simulink model "c_code_MR100"  (R2023a)
settings: Solver=FixedStepAuto  StartTime=0.0  StopTime=10  FixedStep=0.01  MaxStep=0.01  RelTol=1e-3
settings Model: Creator=LJL  LastModifiedBy=LJL
settings OptimizationCC: DefaultParameterBehavior=Inlined  UseDivisionForNetSlopeComputation=on  GainParamInheritBuiltInType=on  UseFloatMulNetSlope=on  InlineInvariantSignals=on  EnhancedBackFolding=on  BooleansAsBitfields=on  PassReuseOutputArgsAs=Individual arguments  StateBitsets=on  DataBitsets=on  ZeroExternalMemoryAtStartup=off  ZeroInternalMemoryAtStartup=off  NoFixptDivByZeroProtection=on  EfficientFloat2IntCast=on  LifeSpan=1  OptimizeBlockOrder=speed  DifferentSizesBufferReuse=on  EfficientTunableParamExpr=on
settings DebuggingCC: ParameterTunabilityLossMsg=error
settings HardwareCC: ProdBitPerInt=16  ProdBitPerPointer=16  ProdBitPerSizeT=16  ProdBitPerPtrDiffT=16  ProdLargestAtomicFloat=None  ProdWordSize=16  ProdLongLongMode=on  ProdHWDeviceType=STMicroelectronics->ST10/Super10
settings SFSimCC: MATLABDynamicMemAlloc=off
settings RTWCC: Description=Embedded Coder  SystemTargetFile=ert.tlc  PackageGeneratedCodeAndArtifacts=on  TemplateMakefile=ert_default_tmf  GenerateReport=on  IncludeHyperlinkInReport=on  LaunchReport=on  GenerateTraceInfo=on  GenerateTraceReport=on  GenerateTraceReportSl=on  GenerateWebview=on
settings CodeAppCC: ForceParamTrailComments=on  IgnoreCustomStorageClasses=off  OperatorAnnotations=on  SimulinkDataObjDesc=on  SFDataObjDesc=on  CustomSymbolStrGlobalVar=rt$N$M  CustomSymbolStrType=$N$M  CustomSymbolStrFcn=$N$M$F  CustomSymbolStrMacro=$N$M  InsertBlockDesc=on
settings ERTTargetCC: TargetLangStandard=C99 (ISO)  GenerateSampleERTMain=on  IncludeMdlTerminateFcn=off  CombineSignalStateStructs=on  SupportComplex=off  SupportContinuousTime=on  InlinedParameterPlacement=NonHierarchical  ERTCustomFileTemplate=example_file_process.tlc  ERTFilePackagingFormat=CompactWithDataFile

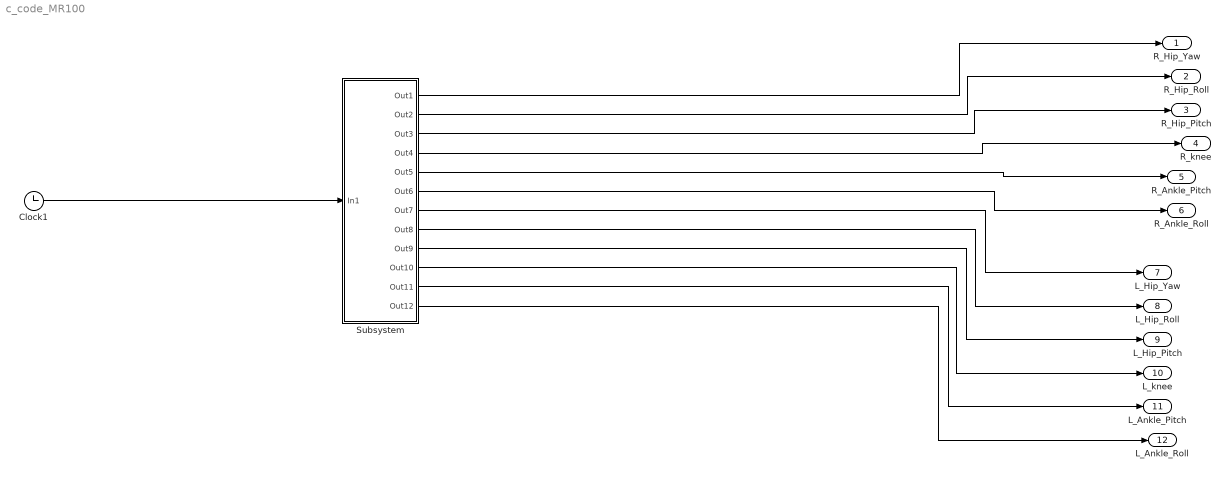
== system c_code_MR100 ==
  Clock1 : Clock
      settings: Decimation=5
  Subsystem : Subsystem
  R_Hip_Yaw : Outport
  R_Hip_Roll : Outport  Port=2
  R_Hip_Pitch : Outport  Port=3
  R_knee : Outport  Port=4
  R_Ankle_Pitch : Outport  Port=5
  R_Ankle_Roll : Outport  Port=6
  L_Hip_Yaw : Outport  Port=7
  L_Hip_Roll : Outport  Port=8
  L_Hip_Pitch : Outport  Port=9
  L_knee : Outport  Port=10
  L_Ankle_Pitch : Outport  Port=11
  L_Ankle_Roll : Outport  Port=12
  wires:
  Clock1/1 -> Subsystem/1(In1)
  Subsystem/1(Out1) -> R_Hip_Yaw/1
  Subsystem/2(Out2) -> R_Hip_Roll/1
  Subsystem/3(Out3) -> R_Hip_Pitch/1
  Subsystem/4(Out4) -> R_knee/1
  Subsystem/5(Out5) -> R_Ankle_Pitch/1
  Subsystem/6(Out6) -> R_Ankle_Roll/1
  Subsystem/7(Out7) -> L_Hip_Yaw/1
  Subsystem/8(Out8) -> L_Hip_Roll/1
  Subsystem/9(Out9) -> L_Hip_Pitch/1
  Subsystem/10(Out10) -> L_knee/1
  Subsystem/11(Out11) -> L_Ankle_Pitch/1
  Subsystem/12(Out12) -> L_Ankle_Roll/1

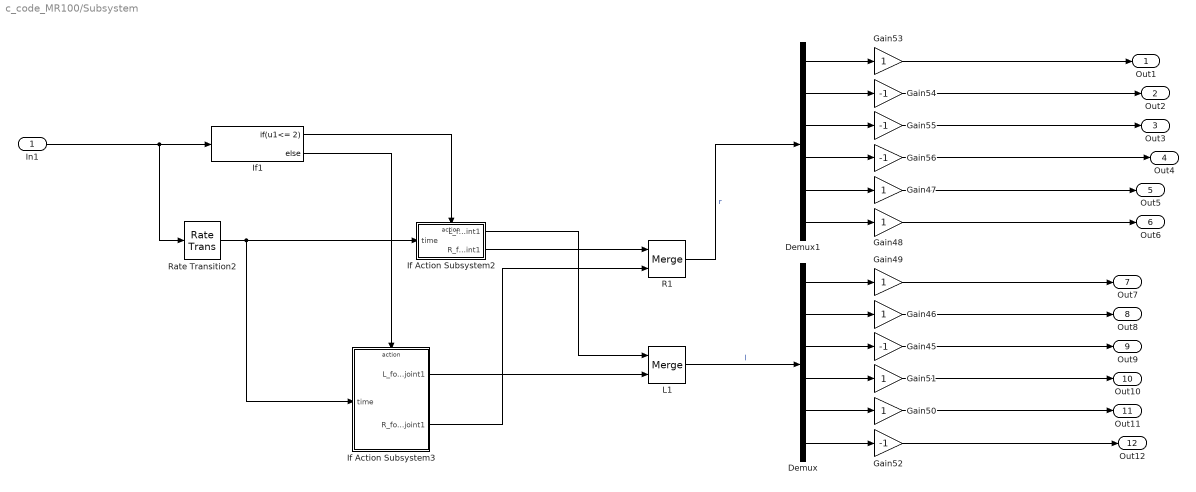
== system c_code_MR100/Subsystem ==
  In1 : Inport
  Demux : Demux  Outputs=6
  Demux1 : Demux  Outputs=6
  Gain{45,52,54..56} (5 alike) : Gain  Gain=-1
  Gain{46..51,53} (7 alike) : Gain
  If Action Subsystem2 : Subsystem  TreatAsAtomicUnit=on
  If Action Subsystem3 : Subsystem  TreatAsAtomicUnit=on
  If1 : If  IfExpression=u1<= 2
  L1 : Merge
  R1 : Merge
  Rate Transition2 : RateTransition  OutPortSampleTime=0.01
  Out1 : Outport
  Out2 : Outport  Port=2
  Out3 : Outport  Port=3
  Out4 : Outport  Port=4
  Out5 : Outport  Port=5
  Out6 : Outport  Port=6
  Out7 : Outport  Port=7
  Out8 : Outport  Port=8
  Out9 : Outport  Port=9
  Out10 : Outport  Port=10
  Out11 : Outport  Port=11
  Out12 : Outport  Port=12
  wires:
  Demux/1 -> Gain49/1
  Demux1/2 -> Gain54/1
  If Action Subsystem2/2(R_foot_joint1) -> R1/1
  Gain52/1 -> Out12/1
  Demux/4 -> Gain51/1
  Demux/6 -> Gain52/1
  Demux/5 -> Gain50/1
  In1/1 -> Rate Transition2/1, If1/1
  If Action Subsystem3/2(R_foot_joint1) -> R1/2
  Rate Transition2/1 -> If Action Subsystem3/1(time), If Action Subsystem2/1(time)
  Demux/2 -> Gain46/1
  If Action Subsystem2/1(L_foot_joint1) -> L1/1
  Demux/3 -> Gain45/1
  Gain46/1 -> Out8/1
  Demux1/3 -> Gain55/1
  Demux1/4 -> Gain56/1
  L1/1 -> Demux/1  "l"
  If1/1 -> If Action Subsystem2/Action
  Demux1/1 -> Gain53/1
  Gain50/1 -> Out11/1
  Demux1/5 -> Gain47/1
  Gain48/1 -> Out6/1
  Demux1/6 -> Gain48/1
  R1/1 -> Demux1/1  "r"
  Gain55/1 -> Out3/1
  If1/2 -> If Action Subsystem3/Action
  Gain54/1 -> Out2/1
  If Action Subsystem3/1(L_foot_joint1) -> L1/2
  Gain56/1 -> Out4/1
  Gain51/1 -> Out10/1
  Gain53/1 -> Out1/1
  Gain47/1 -> Out5/1
  Gain49/1 -> Out7/1
  Gain45/1 -> Out9/1

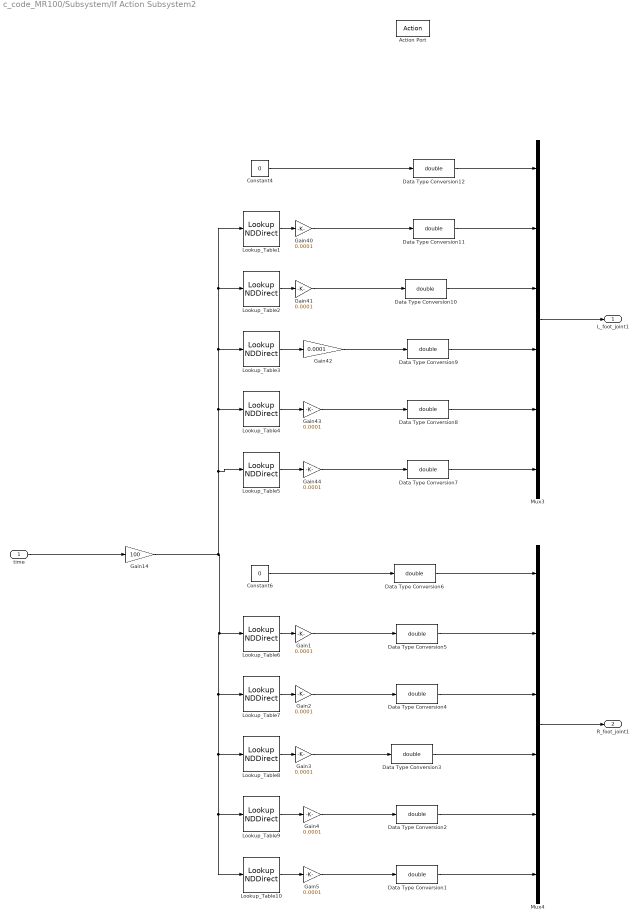
== system c_code_MR100/Subsystem/If Action Subsystem2 ==
  time : Inport
  Action Port : ActionPort  ActionPortLabel=if(u1<= 2)
  Constant4 : Constant  Value=0  SampleTime=-1
  Constant6 : Constant  Value=0  SampleTime=-1
  Data Type Conversion{1..12} (12 alike) : DataTypeConversion  OutDataTypeStr=double  SaturateOnIntegerOverflow=off  RndMeth=Floor
  Gain{1..5,40..44} (10 alike) : Gain  Gain=0.0001
  Gain14 : Gain  Gain=100
  Lookup_Table1 : LookupNDDirect  NumberOfTableDimensions=1  Table=[0;0;0;0;0;0;0;0;0;0;0;0;0;0;0;0;0;0;0;0;0;0;0;0;0;0;0;0;0;0;0;0;0;0;0;0;0;0;0;0;0;0;0;0;0;0;0;0;0;0;0;0;0;0;0;0;0;0;0;0;0;0;0;0;0;0;0;0;0;0;0;0;0;0;0;0;0;0;0;0;0;0;0;0;0;0;0;0;0;0;0;0;0;0;0;0;0;0;0;0;0;0;0;0;0;-1;-1;-2;-4;-6;-9;-12;-17;-22;-29;-37;-46;-57;-69;-83;-99;-117;-137;-159;-183;-209;-238;-269;-303;-339;-378;-420;-463;-510;-559;-610;-664;-720;-779;-839;-902;-966;-1032;-1100;-1169;-1238;-1309;-1380;-1451;-1523;-1593;-1664;-1733;-1802;-1873;-1945;-2018;-2091;-2165;-2238;-2311;-2382;-2452;-2519;-2584;-2644;-2700;-2751;-2795;-2832;-2861;-2882;-2892;-2892;-2881;-2857;-2824;-2781;-2725;-2658;-2580;-2493;-2397;-2294;-2183;-2067;-1946;-1821;-1693;-1562;-1428;-1293;-1157;-1020;-882;-744;-605;-466;-327;-187;-47]  RemoveProtectionInput=on  TableDataTypeStr=int16
  Lookup_Table10 : LookupNDDirect  NumberOfTableDimensions=1  Table=[0;0;0;0;0;0;0;0;0;0;0;0;0;0;0;0;0;0;0;0;0;0;0;0;0;0;0;0;0;0;0;0;0;0;0;0;0;0;0;0;0;0;0;0;0;0;0;0;0;0;0;0;0;0;0;0;0;0;0;0;0;0;0;0;0;0;0;0;0;0;0;0;0;0;0;0;0;0;0;0;0;0;0;0;0;0;0;0;0;0;0;0;0;0;0;0;0;0;0;0;0;0;0;0;0;1;1;2;4;6;9;12;17;22;29;37;46;57;69;83;99;117;137;159;183;209;238;269;303;339;378;420;463;510;559;610;664;720;779;839;902;966;1032;1100;1169;1238;1309;1380;1451;1523;1593;1664;1733;1801;1867;1931;1993;2053;2110;2163;2214;2260;2303;2342;2377;2407;2433;2454;2470;2481;2486;2486;2481;2470;2453;2430;2401;2367;2326;2279;2226;2166;2101;2029;1951;1867;1777;1682;1581;1474;1362;1246;1124;999;870;738;603;466;327;187;47]  RemoveProtectionInput=on  TableDataTypeStr=int16
  Lookup_Table2 : LookupNDDirect  NumberOfTableDimensions=1  Table=[0;0;0;0;0;0;0;0;0;0;0;0;0;0;0;0;0;0;0;0;0;0;0;0;0;0;0;0;0;0;0;0;0;0;0;0;0;0;0;0;0;0;0;0;0;0;0;0;0;0;223;277;396;536;683;832;981;1128;1274;1418;1560;1699;1837;1971;2103;2233;2360;2484;2606;2724;2840;2953;3063;3170;3273;3374;3472;3566;3657;3745;3830;3911;3989;4063;4134;4201;4264;4324;4380;4432;4480;4524;4564;4600;4631;4658;4681;4698;4711;4719;4719;4719;4719;4719;4719;4719;4719;4719;4719;4719;4719;4719;4719;4719;4719;4719;4719;4719;4719;4719;4718;4718;4718;4717;4717;4716;4716;4715;4713;4712;4710;4708;4706;4703;4700;4696;4692;4687;4682;4676;4669;4662;4654;4645;4635;4624;4613;4601;4588;4574;4560;4545;4530;4524;4538;4568;4614;4671;4739;4816;4898;4984;5072;5161;5249;5335;5418;5495;5567;5633;5692;5742;5783;5815;5835;5845;5848;5846;5830;5803;5766;5719;5663;5599;5529;5452;5372;5287;5201;5114;5029;4946;4869;4799;4738;4689;4655;4637;4638;4648;4655]  RemoveProtectionInput=on  TableDataTypeStr=int16
  Lookup_Table3 : LookupNDDirect  NumberOfTableDimensions=1  Table=[0;0;0;0;0;0;0;0;0;0;0;0;0;0;0;0;0;0;0;0;0;0;0;0;0;0;0;0;0;0;0;0;0;0;0;0;0;0;0;0;0;0;0;0;0;0;0;0;0;0;552;688;983;1332;1697;2067;2437;2805;3169;3528;3883;4233;4578;4917;5250;5577;5899;6214;6523;6826;7123;7412;7695;7972;8241;8503;8758;9005;9244;9476;9700;9916;10123;10322;10511;10692;10864;11026;11178;11320;11452;11573;11683;11781;11868;11943;12005;12054;12090;12112;12112;12112;12112;12112;12112;12112;12112;12112;12112;12112;12112;12112;12112;12112;12112;12112;12112;12112;12111;12111;12110;12110;12109;12108;12106;12105;12103;12100;12097;12093;12088;12082;12076;12068;12059;12049;12037;12024;12009;11992;11974;11953;11930;11905;11878;11849;11817;11784;11748;11711;11671;11631;11588;11573;11611;11694;11819;11980;12169;12382;12614;12858;13110;13366;13622;13873;14117;14349;14566;14766;14944;15100;15228;15326;15392;15420;15432;15424;15376;15291;15174;15028;14856;14662;14449;14221;13981;13733;13482;13231;12986;12751;12532;12335;12165;12029;11933;11884;11887;11914;11934]  RemoveProtectionInput=on  TableDataTypeStr=int16
  Lookup_Table4 : LookupNDDirect  NumberOfTableDimensions=1  Table=[0;0;0;0;0;0;0;0;0;0;0;0;0;0;0;0;0;0;0;0;0;0;0;0;0;0;0;0;0;0;0;0;0;0;0;0;0;0;0;0;0;0;0;0;0;0;0;0;0;0;330;411;587;795;1014;1235;1456;1676;1895;2110;2323;2534;2741;2945;3146;3344;3539;3730;3918;4102;4283;4460;4633;4802;4967;5129;5286;5439;5587;5731;5870;6005;6134;6259;6378;6491;6599;6702;6798;6888;6972;7048;7119;7181;7237;7285;7324;7356;7379;7393;7393;7393;7393;7393;7393;7393;7393;7393;7393;7393;7393;7393;7393;7393;7393;7393;7393;7393;7393;7392;7392;7392;7391;7390;7389;7388;7387;7385;7383;7381;7378;7374;7370;7365;7359;7353;7345;7337;7327;7316;7304;7291;7277;7261;7243;7225;7204;7183;7160;7136;7111;7085;7059;7049;7073;7126;7206;7308;7430;7567;7716;7874;8038;8205;8373;8538;8699;8853;8998;9132;9253;9358;9445;9512;9556;9576;9584;9578;9545;9488;9408;9309;9193;9063;8920;8768;8609;8446;8281;8117;7957;7805;7663;7536;7427;7340;7278;7247;7249;7266;7279]  RemoveProtectionInput=on  TableDataTypeStr=int16
  Lookup_Table5 : LookupNDDirect  NumberOfTableDimensions=1  Table=[0;0;0;0;0;0;0;0;0;0;0;0;0;0;0;0;0;0;0;0;0;0;0;0;0;0;0;0;0;0;0;0;0;0;0;0;0;0;0;0;0;0;0;0;0;0;0;0;0;0;0;0;0;0;0;0;0;0;0;0;0;0;0;0;0;0;0;0;0;0;0;0;0;0;0;0;0;0;0;0;0;0;0;0;0;0;0;0;0;0;0;0;0;0;0;0;0;0;0;0;0;0;0;0;0;1;1;2;4;6;9;12;17;22;29;37;46;57;69;83;99;117;137;159;183;209;238;269;303;339;378;420;463;510;559;610;664;720;779;839;902;966;1032;1100;1169;1238;1309;1380;1451;1523;1593;1664;1733;1802;1873;1945;2018;2091;2165;2238;2311;2382;2452;2519;2584;2644;2700;2751;2795;2832;2861;2882;2892;2892;2881;2857;2824;2781;2725;2658;2580;2493;2397;2294;2183;2067;1946;1821;1693;1562;1428;1293;1157;1020;882;744;605;466;327;187;47]  RemoveProtectionInput=on  TableDataTypeStr=int16
  Lookup_Table6 : LookupNDDirect  NumberOfTableDimensions=1  Table=[0;0;0;0;0;0;0;0;0;0;0;0;0;0;0;0;0;0;0;0;0;0;0;0;0;0;0;0;0;0;0;0;0;0;0;0;0;0;0;0;0;0;0;0;0;0;0;0;0;0;0;0;0;0;0;0;0;0;0;0;0;0;0;0;0;0;0;0;0;0;0;0;0;0;0;0;0;0;0;0;0;0;0;0;0;0;0;0;0;0;0;0;0;0;0;0;0;0;0;0;0;0;0;0;0;-1;-1;-2;-4;-6;-9;-12;-17;-22;-29;-37;-46;-57;-69;-83;-99;-117;-137;-159;-183;-209;-238;-269;-303;-339;-378;-420;-463;-510;-559;-610;-664;-720;-779;-839;-902;-966;-1032;-1100;-1169;-1238;-1309;-1380;-1451;-1523;-1593;-1664;-1733;-1801;-1867;-1931;-1993;-2053;-2110;-2163;-2214;-2260;-2303;-2342;-2377;-2407;-2433;-2454;-2470;-2481;-2486;-2486;-2481;-2470;-2453;-2430;-2401;-2367;-2326;-2279;-2226;-2166;-2101;-2029;-1951;-1867;-1777;-1682;-1581;-1474;-1362;-1246;-1124;-999;-870;-738;-603;-466;-327;-187;-47]  RemoveProtectionInput=on  TableDataTypeStr=int16
  Lookup_Table7 : LookupNDDirect  NumberOfTableDimensions=1  Table=[0;0;0;0;0;0;0;0;0;0;0;0;0;0;0;0;0;0;0;0;0;0;0;0;0;0;0;0;0;0;0;0;0;0;0;0;0;0;0;0;0;0;0;0;0;0;0;0;0;0;223;277;396;536;683;832;981;1128;1274;1418;1560;1699;1837;1971;2103;2233;2360;2484;2606;2724;2840;2953;3063;3170;3273;3374;3472;3566;3657;3745;3830;3911;3989;4063;4134;4201;4264;4324;4380;4432;4480;4524;4564;4600;4631;4658;4681;4698;4711;4719;4719;4719;4719;4719;4719;4719;4719;4719;4719;4719;4719;4719;4719;4719;4719;4719;4719;4719;4719;4719;4718;4718;4718;4717;4717;4716;4716;4715;4713;4712;4710;4708;4706;4703;4700;4696;4692;4687;4682;4676;4669;4662;4654;4645;4635;4624;4613;4601;4588;4574;4560;4545;4530;4514;4498;4482;4466;4449;4433;4418;4403;4388;4375;4362;4350;4340;4331;4324;4319;4315;4313;4312;4314;4318;4323;4331;4340;4352;4365;4379;4395;4412;4430;4449;4469;4489;4509;4529;4549;4568;4586;4603;4618;4632;4644;4654;4661;4666;4669;4669;4667]  RemoveProtectionInput=on  TableDataTypeStr=int16
  Lookup_Table8 : LookupNDDirect  NumberOfTableDimensions=1  Table=[0;0;0;0;0;0;0;0;0;0;0;0;0;0;0;0;0;0;0;0;0;0;0;0;0;0;0;0;0;0;0;0;0;0;0;0;0;0;0;0;0;0;0;0;0;0;0;0;0;0;552;688;983;1332;1697;2067;2437;2805;3169;3528;3883;4233;4578;4917;5250;5577;5899;6214;6523;6826;7123;7412;7695;7972;8241;8503;8758;9005;9244;9476;9700;9916;10123;10322;10511;10692;10864;11026;11178;11320;11452;11573;11683;11781;11868;11943;12005;12054;12090;12112;12112;12112;12112;12112;12112;12112;12112;12112;12112;12112;12112;12112;12112;12112;12112;12112;12112;12112;12111;12111;12110;12110;12109;12108;12106;12105;12103;12100;12097;12093;12088;12082;12076;12068;12059;12049;12037;12024;12009;11992;11974;11953;11930;11905;11878;11849;11817;11784;11748;11711;11671;11631;11588;11545;11501;11457;11412;11368;11324;11281;11240;11200;11163;11129;11098;11070;11046;11026;11011;11000;10995;10994;10999;11009;11024;11045;11070;11101;11136;11175;11218;11265;11315;11367;11421;11476;11531;11586;11640;11693;11743;11789;11832;11870;11903;11930;11951;11966;11973;11973;11966]  RemoveProtectionInput=on  TableDataTypeStr=int16
  Lookup_Table9 : LookupNDDirect  NumberOfTableDimensions=1  Table=[0;0;0;0;0;0;0;0;0;0;0;0;0;0;0;0;0;0;0;0;0;0;0;0;0;0;0;0;0;0;0;0;0;0;0;0;0;0;0;0;0;0;0;0;0;0;0;0;0;0;330;411;587;795;1014;1235;1456;1676;1895;2110;2323;2534;2741;2945;3146;3344;3539;3730;3918;4102;4283;4460;4633;4802;4967;5129;5286;5439;5587;5731;5870;6005;6134;6259;6378;6491;6599;6702;6798;6888;6972;7048;7119;7181;7237;7285;7324;7356;7379;7393;7393;7393;7393;7393;7393;7393;7393;7393;7393;7393;7393;7393;7393;7393;7393;7393;7393;7393;7393;7392;7392;7392;7391;7390;7389;7388;7387;7385;7383;7381;7378;7374;7370;7365;7359;7353;7345;7337;7327;7316;7304;7291;7277;7261;7243;7225;7204;7183;7160;7136;7111;7085;7059;7031;7003;6975;6946;6918;6890;6863;6837;6812;6789;6767;6747;6730;6714;6702;6692;6686;6682;6682;6685;6691;6701;6714;6730;6749;6771;6796;6824;6853;6885;6918;6952;6987;7022;7057;7092;7125;7157;7187;7214;7238;7259;7277;7290;7299;7304;7304;7300]  RemoveProtectionInput=on  TableDataTypeStr=int16
  Mux3 : Mux  Inputs=6
  Mux4 : Mux  Inputs=6
  L_foot_joint1 : Outport
  R_foot_joint1 : Outport  Port=2
  wires:
  Constant4/1 -> Data Type Conversion12/1
  Lookup_Table4/1 -> Gain43/1
  Lookup_Table3/1 -> Gain42/1
  Lookup_Table5/1 -> Gain44/1
  Lookup_Table1/1 -> Gain40/1
  time/1 -> Gain14/1
  Lookup_Table2/1 -> Gain41/1
  Mux3/1 -> L_foot_joint1/1
  Gain43/1 -> Data Type Conversion8/1
  Gain42/1 -> Data Type Conversion9/1
  Gain44/1 -> Data Type Conversion7/1
  Gain41/1 -> Data Type Conversion10/1
  Gain40/1 -> Data Type Conversion11/1
  Gain1/1 -> Data Type Conversion5/1
  Gain2/1 -> Data Type Conversion4/1
  Lookup_Table7/1 -> Gain2/1
  Gain5/1 -> Data Type Conversion1/1
  Lookup_Table9/1 -> Gain4/1
  Lookup_Table6/1 -> Gain1/1
  Lookup_Table10/1 -> Gain5/1
  Lookup_Table8/1 -> Gain3/1
  Gain3/1 -> Data Type Conversion3/1
  Gain4/1 -> Data Type Conversion2/1
  Mux4/1 -> R_foot_joint1/1
  Gain14/1 -> Lookup_Table7/1, Lookup_Table8/1, Lookup_Table9/1, Lookup_Table10/1, Lookup_Table6/1, Lookup_Table5/1, Lookup_Table1/1, Lookup_Table2/1, Lookup_Table3/1, Lookup_Table4/1
  Constant6/1 -> Data Type Conversion6/1
  Data Type Conversion1/1 -> Mux4/6
  Data Type Conversion2/1 -> Mux4/5
  Data Type Conversion3/1 -> Mux4/4
  Data Type Conversion4/1 -> Mux4/3
  Data Type Conversion5/1 -> Mux4/2
  Data Type Conversion6/1 -> Mux4/1
  Data Type Conversion7/1 -> Mux3/6
  Data Type Conversion8/1 -> Mux3/5
  Data Type Conversion9/1 -> Mux3/4
  Data Type Conversion10/1 -> Mux3/3
  Data Type Conversion11/1 -> Mux3/2
  Data Type Conversion12/1 -> Mux3/1

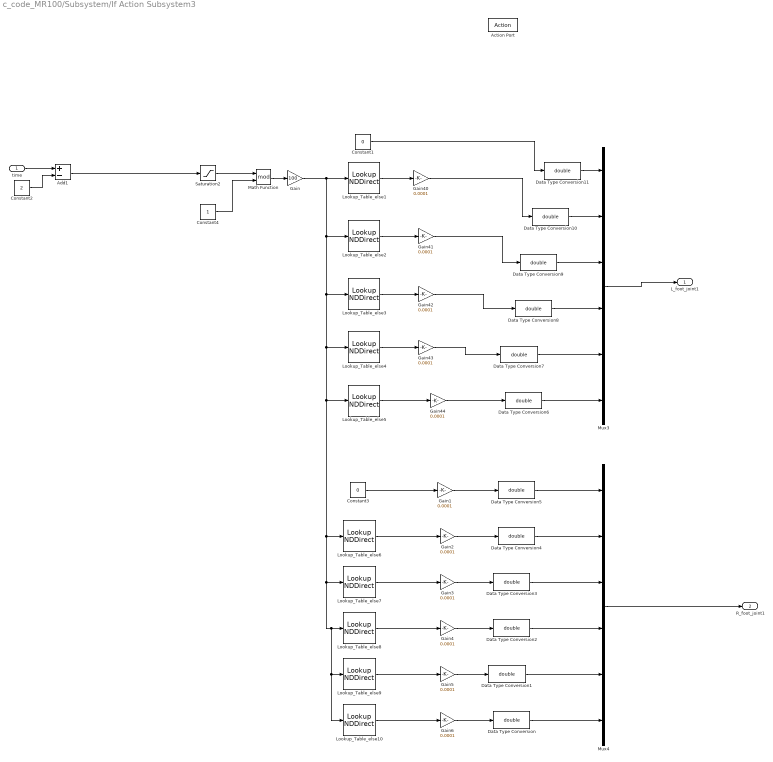
== system c_code_MR100/Subsystem/If Action Subsystem3 ==
  time : Inport
  Action Port : ActionPort  ActionPortLabel=else
  Add1 : Sum  Inputs=+-
  Constant1 : Constant  Value=0  SampleTime=-1
  Constant2 : Constant  Value=2
  Constant3 : Constant  Value=0  SampleTime=-1
  Constant4 : Constant
  Data Type Conversion{,1..11} (12 alike) : DataTypeConversion  OutDataTypeStr=double  SaturateOnIntegerOverflow=off  RndMeth=Floor
  Gain : Gain  Gain=100
  Gain{1..6,40..44} (11 alike) : Gain  Gain=0.0001
  Lookup_Table_else1 : LookupNDDirect  NumberOfTableDimensions=1  Table=[93;232;369;505;638;767;893;1014;1131;1242;1348;1448;1541;1628;1709;1782;1848;1907;1958;2002;2038;2066;2086;2099;2104;2101;2090;2071;2044;2010;1968;1918;1861;1797;1725;1646;1561;1469;1370;1266;1156;1041;922;798;670;539;406;270;133;-4;-142;-279;-414;-550;-684;-817;-949;-1079;-1208;-1334;-1458;-1578;-1694;-1806;-1912;-2013;-2107;-2192;-2270;-2337;-2395;-2440;-2474;-2495;-2502;-2497;-2481;-2450;-2407;-2351;-2284;-2207;-2120;-2026;-1924;-1816;-1702;-1584;-1462;-1337;-1210;-1080;-948;-816;-682;-547;-412;-275;-138;0]  RemoveProtectionInput=on  TableDataTypeStr=int16
  Lookup_Table_else10 : LookupNDDirect  NumberOfTableDimensions=1  Table=[-93;-232;-370;-507;-642;-777;-910;-1041;-1171;-1298;-1422;-1543;-1661;-1773;-1881;-1982;-2076;-2163;-2241;-2310;-2368;-2414;-2449;-2470;-2478;-2475;-2459;-2430;-2388;-2333;-2267;-2190;-2105;-2011;-1910;-1803;-1690;-1573;-1452;-1328;-1201;-1072;-941;-809;-675;-541;-406;-270;-133;4;142;279;414;548;679;807;931;1051;1166;1277;1381;1480;1573;1659;1738;1810;1875;1933;1983;2026;2061;2089;2108;2120;2124;2120;2108;2088;2061;2026;1983;1933;1875;1809;1737;1658;1572;1479;1380;1275;1165;1049;929;805;676;545;411;275;138;0]  RemoveProtectionInput=on  TableDataTypeStr=int16
  Lookup_Table_else2 : LookupNDDirect  NumberOfTableDimensions=1  Table=[4660;4662;4662;4659;4654;4647;4637;4627;4614;4601;4586;4571;4555;4540;4524;4509;4495;4482;4470;4460;4451;4444;4439;4436;4435;4436;4439;4444;4451;4460;4471;4483;4497;4511;4527;4543;4559;4575;4591;4606;4620;4634;4645;4656;4664;4670;4674;4675;4674;4671;4665;4656;4655;4673;4706;4754;4813;4881;4958;5039;5125;5212;5300;5386;5470;5551;5626;5696;5760;5815;5863;5901;5930;5947;5953;5952;5945;5926;5894;5852;5799;5738;5668;5592;5509;5422;5331;5239;5146;5054;4965;4883;4807;4743;4690;4653;4634;4634;4643;4650]  RemoveProtectionInput=on  TableDataTypeStr=int16
  Lookup_Table_else3 : LookupNDDirect  NumberOfTableDimensions=1  Table=[11948;11954;11953;11945;11931;11911;11885;11855;11821;11783;11743;11701;11659;11616;11573;11532;11493;11457;11424;11396;11372;11353;11339;11330;11328;11331;11339;11354;11373;11398;11427;11461;11498;11538;11580;11624;11668;11713;11757;11799;11838;11875;11908;11936;11958;11975;11986;11990;11987;11978;11961;11937;11935;11984;12077;12209;12374;12567;12783;13016;13261;13514;13769;14024;14274;14516;14745;14959;15155;15329;15478;15599;15690;15745;15763;15762;15741;15677;15577;15442;15278;15087;14873;14639;14390;14130;13862;13591;13321;13057;12805;12571;12359;12178;12032;11929;11875;11875;11902;11921]  RemoveProtectionInput=on  TableDataTypeStr=int16
  Lookup_Table_else4 : LookupNDDirect  NumberOfTableDimensions=1  Table=[7288;7292;7291;7286;7277;7264;7248;7229;7207;7183;7157;7131;7103;7076;7049;7023;6998;6975;6954;6936;6921;6909;6900;6895;6893;6895;6900;6909;6922;6938;6956;6977;7001;7026;7053;7081;7109;7138;7166;7193;7218;7241;7262;7280;7295;7305;7312;7315;7313;7307;7296;7281;7280;7311;7370;7455;7561;7686;7825;7976;8136;8301;8470;8638;8804;8965;9119;9263;9395;9513;9615;9698;9760;9798;9811;9810;9795;9752;9683;9591;9479;9349;9204;9048;8881;8708;8531;8352;8175;8003;7840;7688;7552;7435;7342;7276;7241;7242;7258;7271]  RemoveProtectionInput=on  TableDataTypeStr=int16
  Lookup_Table_else5 : LookupNDDirect  NumberOfTableDimensions=1  Table=[-93;-232;-369;-505;-638;-767;-893;-1014;-1131;-1242;-1348;-1448;-1541;-1628;-1709;-1782;-1848;-1907;-1958;-2002;-2038;-2066;-2086;-2099;-2104;-2101;-2090;-2071;-2044;-2010;-1968;-1918;-1861;-1797;-1725;-1646;-1561;-1469;-1370;-1266;-1156;-1041;-922;-798;-670;-539;-406;-270;-133;4;142;279;414;550;684;817;949;1079;1208;1334;1458;1578;1694;1806;1912;2013;2107;2192;2270;2337;2395;2440;2474;2495;2502;2497;2481;2450;2407;2351;2284;2207;2120;2026;1924;1816;1702;1584;1462;1337;1210;1080;948;816;682;547;412;275;138;0]  RemoveProtectionInput=on  TableDataTypeStr=int16
  Lookup_Table_else6 : LookupNDDirect  NumberOfTableDimensions=1  Table=[93;232;370;507;642;777;910;1041;1171;1298;1422;1543;1661;1773;1881;1982;2076;2163;2241;2310;2368;2414;2449;2470;2478;2475;2459;2430;2388;2333;2267;2190;2105;2011;1910;1803;1690;1573;1452;1328;1201;1072;941;809;675;541;406;270;133;-4;-142;-279;-414;-548;-679;-807;-931;-1051;-1166;-1277;-1381;-1480;-1573;-1659;-1738;-1810;-1875;-1933;-1983;-2026;-2061;-2089;-2108;-2120;-2124;-2120;-2108;-2088;-2061;-2026;-1983;-1933;-1875;-1809;-1737;-1658;-1572;-1479;-1380;-1275;-1165;-1049;-929;-805;-676;-545;-411;-275;-138;0]  RemoveProtectionInput=on  TableDataTypeStr=int16
  Lookup_Table_else7 : LookupNDDirect  NumberOfTableDimensions=1  Table=[4661;4653;4654;4672;4706;4754;4814;4883;4960;5042;5128;5215;5303;5390;5474;5555;5631;5701;5764;5820;5868;5906;5934;5952;5957;5957;5950;5930;5898;5855;5803;5741;5672;5595;5512;5425;5334;5241;5148;5056;4967;4884;4809;4744;4691;4654;4634;4634;4644;4651;4655;4657;4656;4653;4648;4640;4631;4620;4607;4593;4579;4563;4548;4532;4517;4502;4488;4475;4463;4453;4444;4437;4432;4430;4429;4430;4434;4439;4447;4456;4467;4480;4494;4509;4524;4540;4557;4573;4590;4605;4620;4633;4645;4655;4664;4670;4674;4675;4674;4671]  RemoveProtectionInput=on  TableDataTypeStr=int16
  Lookup_Table_else8 : LookupNDDirect  NumberOfTableDimensions=1  Table=[11952;11930;11931;11981;12076;12210;12377;12571;12789;13023;13269;13523;13780;14035;14286;14528;14758;14973;15169;15343;15493;15614;15704;15760;15778;15777;15755;15691;15590;15455;15290;15098;14883;14649;14400;14139;13870;13598;13328;13063;12811;12576;12364;12181;12035;11932;11877;11877;11903;11922;11934;11939;11937;11928;11913;11893;11867;11836;11801;11763;11723;11681;11638;11595;11552;11511;11473;11437;11405;11376;11353;11334;11321;11313;11312;11315;11325;11340;11361;11387;11417;11451;11489;11530;11573;11618;11663;11708;11753;11796;11836;11873;11906;11935;11958;11975;11986;11991;11988;11978]  RemoveProtectionInput=on  TableDataTypeStr=int16
  Lookup_Table_else9 : LookupNDDirect  NumberOfTableDimensions=1  Table=[7290;7276;7277;7309;7370;7456;7563;7689;7829;7981;8142;8308;8476;8645;8812;8973;9128;9272;9405;9523;9625;9708;9770;9809;9821;9820;9805;9761;9692;9599;9487;9357;9212;9054;8887;8714;8536;8357;8180;8007;7843;7691;7555;7438;7344;7277;7243;7243;7259;7271;7279;7282;7281;7275;7266;7253;7236;7216;7194;7170;7144;7117;7090;7063;7036;7010;6985;6962;6942;6924;6909;6897;6889;6884;6883;6885;6891;6901;6914;6930;6949;6971;6995;7021;7049;7077;7106;7135;7163;7191;7216;7240;7261;7279;7294;7305;7312;7315;7314;7307]  RemoveProtectionInput=on  TableDataTypeStr=int16
  Math Function : Math  Operator=mod
  Mux3 : Mux  Inputs=6
  Mux4 : Mux  Inputs=6
  Saturation2 : Saturate  UpperLimit=inf  LowerLimit=0
  L_foot_joint1 : Outport
  R_foot_joint1 : Outport  Port=2
  wires:
  Lookup_Table_else7/1 -> Gain3/1
  Lookup_Table_else10/1 -> Gain6/1
  Mux3/1 -> L_foot_joint1/1
  Gain44/1 -> Data Type Conversion6/1
  Gain40/1 -> Data Type Conversion10/1
  Gain41/1 -> Data Type Conversion9/1
  Lookup_Table_else3/1 -> Gain42/1
  Gain4/1 -> Data Type Conversion2/1
  Lookup_Table_else1/1 -> Gain40/1
  Gain2/1 -> Data Type Conversion4/1
  Gain6/1 -> Data Type Conversion/1
  Math Function/1 -> Gain/1
  Add1/1 -> Saturation2/1
  Constant4/1 -> Math Function/2
  Gain/1 -> Lookup_Table_else2/1, Lookup_Table_else3/1, Lookup_Table_else4/1, Lookup_Table_else5/1, Lookup_Table_else6/1, Lookup_Table_else7/1, Lookup_Table_else10/1, Lookup_Table_else9/1, Lookup_Table_else8/1, Lookup_Table_else1/1
  Constant2/1 -> Add1/2
  Lookup_Table_else5/1 -> Gain44/1
  Gain3/1 -> Data Type Conversion3/1
  Lookup_Table_else8/1 -> Gain4/1
  time/1 -> Add1/1
  Lookup_Table_else2/1 -> Gain41/1
  Lookup_Table_else9/1 -> Gain5/1
  Saturation2/1 -> Math Function/1
  Constant3/1 -> Gain1/1
  Constant1/1 -> Data Type Conversion11/1
  Gain1/1 -> Data Type Conversion5/1
  Gain5/1 -> Data Type Conversion1/1
  Gain42/1 -> Data Type Conversion8/1
  Lookup_Table_else4/1 -> Gain43/1
  Mux4/1 -> R_foot_joint1/1
  Lookup_Table_else6/1 -> Gain2/1
  Gain43/1 -> Data Type Conversion7/1
  Data Type Conversion/1 -> Mux4/6
  Data Type Conversion1/1 -> Mux4/5
  Data Type Conversion2/1 -> Mux4/4
  Data Type Conversion3/1 -> Mux4/3
  Data Type Conversion4/1 -> Mux4/2
  Data Type Conversion5/1 -> Mux4/1
  Data Type Conversion6/1 -> Mux3/6
  Data Type Conversion7/1 -> Mux3/5
  Data Type Conversion8/1 -> Mux3/4
  Data Type Conversion9/1 -> Mux3/3
  Data Type Conversion10/1 -> Mux3/2
  Data Type Conversion11/1 -> Mux3/1
